simulink model "robot3_model_mob_control3"  (R2023b)
settings: Solver=FixedStepAuto  StartTime=0.0  StopTime=4*pi  RelTol=1e-3
values from neighbouring files (symbols this model uses):
  Ac3 = zeros(n)    [solveP.m]
undefined symbols (not defined in the file or in its folder): Bc3, Cartesian_trajectory, Cc3, Coriolis3, CoriolisT3, Dhat3, Dinv3, Forward_kin3, Gravity3, L3
libraries: simulink x1
settings Model: Creator=사용자  LastModifiedBy=rodel
settings SolverCC: ZeroCrossAlgorithm=Adaptive
settings DebuggingCC: IgnoredZcDiagnostic=none

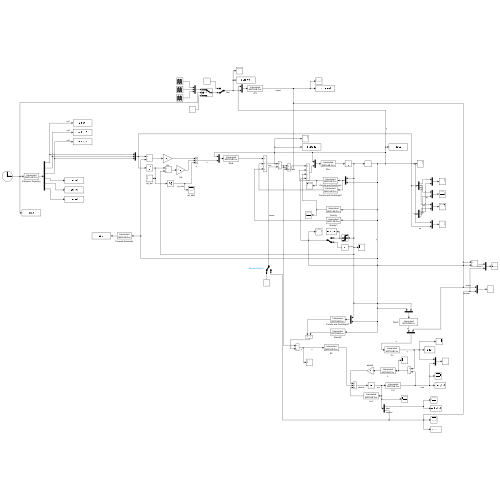
[thumbnail: Simulink's stored preview of the top-level diagram]
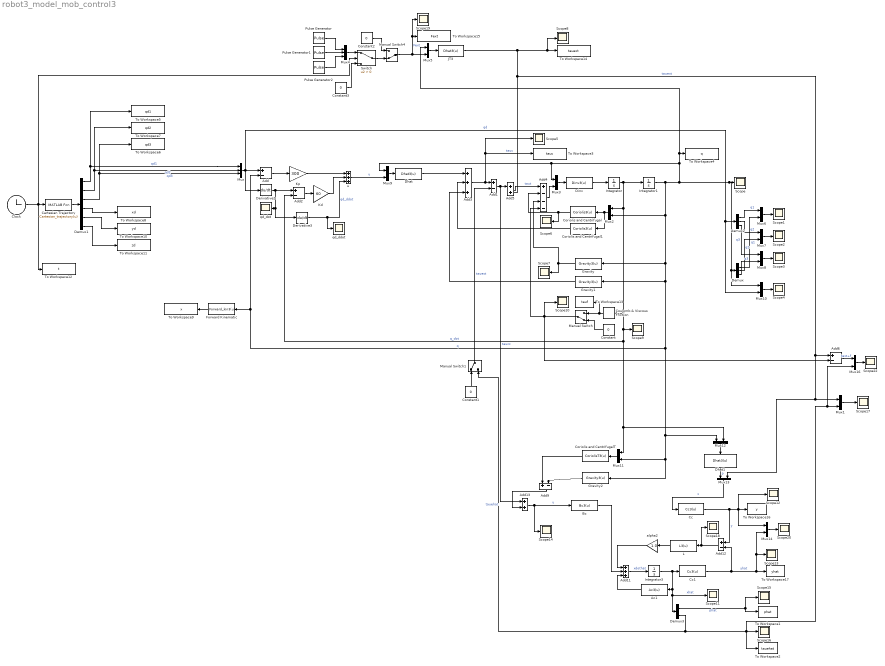
== system robot3_model_mob_control3 ==
  Ac1 : MATLABFcn  MATLABFcn=Ac3(u)  OutputDimensions=6  Output1D=off
  Add{,1..2,6,9,12} (6 alike) : Sum  Inputs=+-
  Add11 : Sum  Inputs=+++
  Add13 : Sum
  Add3 : Sum  Inputs=+++
  Add4 : Sum  Inputs=+---
  Add5 : Sum
  Bc : MATLABFcn  MATLABFcn=Bc3(u)  OutputDimensions=6  Output1D=off
  Cartesian Trajectory : MATLABFcn  MATLABFcn=Cartesian_trajectory(u)  OutputDimensions=6  Output1D=off
  Cc : MATLABFcn  MATLABFcn=Cc3(u)  OutputDimensions=3  Output1D=off
  Cc1 : MATLABFcn  MATLABFcn=Cc3(u)  OutputDimensions=3  Output1D=off
  Clock : Clock
  Constant{,1..3} (4 alike) : Constant  Value=0
  Coriolis and Centrifugal : MATLABFcn  MATLABFcn=Coriolis3(u)  OutputDimensions=3  Output1D=off
  Coriolis and Centrifugal1 : MATLABFcn  MATLABFcn=Coriolis3(u)  OutputDimensions=3  Output1D=off
  Coriolis and CentrifugalT : MATLABFcn  MATLABFcn=CoriolisT3(u)  OutputDimensions=3  Output1D=off
  Coulomb & Viscous Friction : simulink/Discontinuities/Coulomb & Viscous Friction  offset=5  gain=3
  Demux : Demux  Outputs=3
  Demux1 : Demux  Outputs=6
  Demux2 : Demux  Outputs=3
  Demux3 : Demux  Outputs=2
  Derivative2 : Derivative
  Derivative3 : Derivative
  Dhat : MATLABFcn  MATLABFcn=Dhat3(u)  OutputDimensions=3  Output1D=off
  Dhat1 : MATLABFcn  MATLABFcn=Dhat3(u)  OutputDimensions=3  Output1D=off
  Dinv : MATLABFcn  MATLABFcn=Dinv3(u)  OutputDimensions=3  Output1D=off
  Forward Kinematic : MATLABFcn  MATLABFcn=Forward_kin3(u)  OutputDimensions=3  Output1D=off
  Gravity : MATLABFcn  MATLABFcn=Gravity3(u)  OutputDimensions=3  Output1D=off
  Gravity1 : MATLABFcn  MATLABFcn=Gravity3(u)  OutputDimensions=3  Output1D=off
  Gravity2 : MATLABFcn  MATLABFcn=Gravity3(u)  OutputDimensions=3  Output1D=off
  Integrator : Integrator  InitialCondition=[0;0;0];
  Integrator1 : Integrator  InitialCondition=[0.9587;0.7246;-1.1694]
  Integrator3 : Integrator  InitialCondition=[0; 0; 0; 0; 0; 0];
  JT3 : MATLABFcn  MATLABFcn=Dhat3(u)  OutputDimensions=3  Output1D=off
  Kd : Gain  Gain=60
  Kp : Gain  Gain=300
  L : MATLABFcn  MATLABFcn=L3(u)  OutputDimensions=6  Output1D=off
  Manual Switch : ManualSwitch  CurrentSetting=0
  Manual Switch1 : ManualSwitch
  Manual Switch4 : ManualSwitch  CurrentSetting=0
  Mux : Mux  Inputs=3
  Mux{1..3,5..14,16} (14 alike) : Mux  Inputs=2
  Mux4 : Mux  Inputs=3
  Pulse Generator : DiscretePulseGenerator  PulseType=Time based  Amplitude=10  PulseWidth=2  PhaseDelay=2
  Pulse Generator1 : DiscretePulseGenerator  PulseType=Time based  Amplitude=10  PhaseDelay=3
  Pulse Generator2 : DiscretePulseGenerator  PulseType=Time based  Amplitude=50  PulseWidth=80  PhaseDelay=2
  Scope{,1..20,22} (22 alike) : Scope
  Switch : Switch  Criteria=u2 > Threshold  SaturateOnIntegerOverflow=off  InputSameDT=off
  To Workspace1 : ToWorkspace  VariableName=phat  SaveFormat=Timeseries  SampleTime=0.001
  To Workspace10 : ToWorkspace  VariableName=yd  SampleTime=0.001
  To Workspace11 : ToWorkspace  VariableName=zd  SampleTime=0.001
  To Workspace12 : ToWorkspace  VariableName=t  SaveFormat=Timeseries  SampleTime=0.001
  To Workspace13 : ToWorkspace  VariableName=tauf  SaveFormat=Timeseries  SampleTime=0.001
  To Workspace14 : ToWorkspace  VariableName=tauext  SaveFormat=Timeseries  SampleTime=0.001
  To Workspace15 : ToWorkspace  VariableName=Fext  SaveFormat=Timeseries  SampleTime=0.001
  To Workspace16 : ToWorkspace  VariableName=y  SaveFormat=Timeseries  SampleTime=0.001
  To Workspace17 : ToWorkspace  VariableName=yhat  SaveFormat=Timeseries  SampleTime=0.001
  To Workspace2 : ToWorkspace  VariableName=tauehat  SaveFormat=Timeseries  SampleTime=0.001
  To Workspace3 : ToWorkspace  VariableName=tauc  SaveFormat=Timeseries  SampleTime=0.001
  To Workspace4 : ToWorkspace  VariableName=q  SaveFormat=Timeseries  SampleTime=0.001
  To Workspace5 : ToWorkspace  VariableName=qd1  SaveFormat=Timeseries  SampleTime=0.001
  To Workspace6 : ToWorkspace  VariableName=qd3  SaveFormat=Timeseries  SampleTime=0.001
  To Workspace7 : ToWorkspace  VariableName=qd2  SaveFormat=Timeseries  SampleTime=0.001
  To Workspace8 : ToWorkspace  VariableName=xd  SampleTime=0.001
  To Workspace9 : ToWorkspace  VariableName=x  SampleTime=0.001
  alpha2 : Gain  Gain=1.0
  qd_ddot : Scope
  qd_dot : Scope
  u : Sum  Inputs=+++
  wires:
  Mux/1 -> Derivative2/1, Mux10/2, Demux2/1, Add/1  "qd"
  Add2/1 -> Kd/1
  Kp/1 -> u/1
  Kd/1 -> u/2
  Add/1 -> Kp/1
  Dinv/1 -> Integrator/1
  Mux2/1 -> Coriolis and Centrifugal/1, Coriolis and Centrifugal1/1
  Integrator/1 -> Mux11/1, Mux12/2, Add2/2, Scope9/1, Coulomb & Viscous Friction/1, Mux2/1, Integrator1/1  "q_dot"
  Derivative3/1 -> qd_ddot/1, u/3  "qd_ddot"
  Mux9/1 -> Dhat/1
  Mux3/1 -> Dinv/1
  Dhat/1 -> Add3/1
  Coriolis and Centrifugal1/1 -> Add3/2
  Gravity1/1 -> Add3/3
  Coriolis and Centrifugal/1 -> Add4/2, Scope6/1
  Gravity/1 -> Add4/3, Scope7/1
  Constant/1 -> Manual Switch/2
  Coulomb & Viscous Friction/1 -> To Workspace13/1, Manual Switch/1
  Derivative2/1 -> Derivative3/1, qd_dot/1, Add2/1
  Forward Kinematic/1 -> To Workspace9/1
  Demux1/5 -> To Workspace10/1
  Demux1/4 -> To Workspace8/1
  Demux1/3 -> To Workspace6/1, Mux/3  "qd3"
  Cartesian Trajectory/1 -> Demux1/1
  Demux1/1 -> To Workspace5/1, Mux/1  "qd1"
  Demux1/6 -> To Workspace11/1
  Demux1/2 -> Mux/2, To Workspace7/1  "qd2"
  u/1 -> Mux9/2  "u"
  Add3/1 -> Add1/1, Scope5/1, To Workspace3/1  "tauc"
  Demux/2 -> Mux7/2  "q2"
  Mux6/1 -> Scope1/1
  Mux7/1 -> Scope2/1
  Mux8/1 -> Scope3/1
  Demux/1 -> Mux6/2  "q1"
  Demux/3 -> Mux8/2  "q3"
  Mux10/1 -> Scope4/1
  Demux2/1 -> Mux6/1  "q1"
  Demux2/2 -> Mux7/1  "q2"
  Demux2/3 -> Mux8/1  "q3"
  Gravity2/1 -> Add9/2
  Add11/1 -> Integrator3/1  "xdothat"
  Cc/1 -> Mux14/1, To Workspace16/1, Scope12/1, Add12/1  "y"
  Cc1/1 -> Add12/2, Mux14/2, Scope13/1, To Workspace17/1  "yhat"
  Add12/1 -> Scope18/1, L/1
  L/1 -> alpha2/1
  Integrator3/1 -> Demux3/1, Scope11/1, Ac1/1, Cc1/1  "xhat"
  Ac1/1 -> Add11/3
  Mux11/1 -> Coriolis and CentrifugalT/1
  Add9/1 -> Add13/2
  Add4/1 -> Mux3/2
  Add13/1 -> Bc/1, Scope14/1  "u"
  Bc/1 -> Add11/2
  Coriolis and CentrifugalT/1 -> Add9/1
  Demux3/1 -> Scope15/1, To Workspace1/1  "phat"
  Demux3/2 -> Mux1/2, Mux16/2, To Workspace2/1, Scope16/1, Manual Switch1/2  "tauehat"
  Mux1/1 -> Scope17/1
  Add5/1 -> Add4/1  "taut"
  Constant1/1 -> Manual Switch1/1
  Manual Switch/1 -> Scope10/1, Add4/4, Add6/2
  Manual Switch4/1 -> Scope19/1, To Workspace15/1, Mux5/2  "Fext"
  JT3/1 -> Add6/1, Mux13/2, Mux1/1, Add5/2, To Workspace14/1, Scope8/1  "tauext"
  Mux5/1 -> JT3/1
  Switch/1 -> Manual Switch4/2
  Pulse Generator/1 -> Mux4/1
  Constant3/1 -> Switch/3
  Pulse Generator2/1 -> Mux4/3
  Constant2/1 -> Manual Switch4/1
  Clock/1 -> Switch/2, To Workspace12/1, Cartesian Trajectory/1
  Pulse Generator1/1 -> Mux4/2
  Mux4/1 -> Switch/1
  Integrator1/1 -> Mux5/1, To Workspace4/1, Mux3/1, Mux9/1, Mux10/1, Demux/1, Scope/1, Mux2/2, Forward Kinematic/1, Add/2, Mux12/1, Gravity2/1, Mux11/2, Gravity1/1, Gravity/1  "q"
  Manual Switch1/1 -> Add1/2  "tauest"
  Mux12/1 -> Dhat1/1
  Dhat1/1 -> Mux13/1  "p"
  Mux13/1 -> Cc/1  "x"
  alpha2/1 -> Add11/1
  Mux14/1 -> Scope20/1
  Add1/1 -> Add13/1, Add5/1  "taucc"
  Add6/1 -> Mux16/1  "text+f"
  Mux16/1 -> Scope22/1
